simulink model "my_svpwm_controller"  (R2020a)
settings: Solver=VariableStepAuto  StartTime=0.0  StopTime=0.05  FixedStep=10e-6  MaxStep=0.00001  RelTol=1e-3  EnableMultiTasking=on
InitFcn:
  | f = 50;
libraries: dsparch4 x3, simulink x1, powerlib x1
settings Model: Creator=Administrator  LastModifiedBy=DELL
settings DataIOCC: LimitDataPoints=on  SaveFormat=Array  SignalLoggingSaveFormat=ModelDataLogs  ReturnWorkspaceOutputs=off
settings OptimizationCC: ExpressionDepthLimit=2147483647  InitFltsAndDblsToZero=on  LifeSpan=inf
settings DebuggingCC: SaveWithParameterizedLinksMsg=none  UnderspecifiedInitializationDetection=Classic  MergeDetectMultiDrivingBlocksExec=none  SignalResolutionControl=TryResolveAllWithWarning  SolverPrmCheckMsg=warning  MultiTaskDSMMsg=warning  MultiTaskCondExecSysMsg=none  FcnCallInpInsideContextMsg=warning  StateNameClashWarn=warning  SFUnexpectedBacktrackingDiag=warning  SFNoUnconditionalDefaultTransitionDiag=warning  ArithmeticOperatorsInVariantConditions=warning
settings HardwareCC: ProdBitPerPointer=32  ProdBitPerSizeT=32  ProdBitPerPtrDiffT=32  ProdLargestAtomicFloat=None  ProdIntDivRoundTo=Undefined  ProdEndianess=Unspecified  ProdWordSize=32  ProdHWDeviceType=32-bit Generic
settings ModelReferenceCC: PropagateSignalLabelsOutOfModel=off
settings SFSimCC: SimUseLocalCustomCode=off  CustomCodeUndefinedFunction=UseInterfaceOnly
settings RTWCC: RTWUseLocalCustomCode=off
settings CodeAppCC: StateflowObjectComments=on
settings GRTTargetCC: TargetFcnLib=ansi_tfl_tmw.mat  TargetLangStandard=C89/C90 (ANSI)  CombineOutputUpdateFcns=off  GRTInterface=on
settings ConfigComp: CovMetricSettings=dw  CovHtmlReporting=on  CovSaveCumulativeToWorkspaceVar=on  CovSaveSingleToWorkspaceVar=on  CovExternalEMLEnable=off

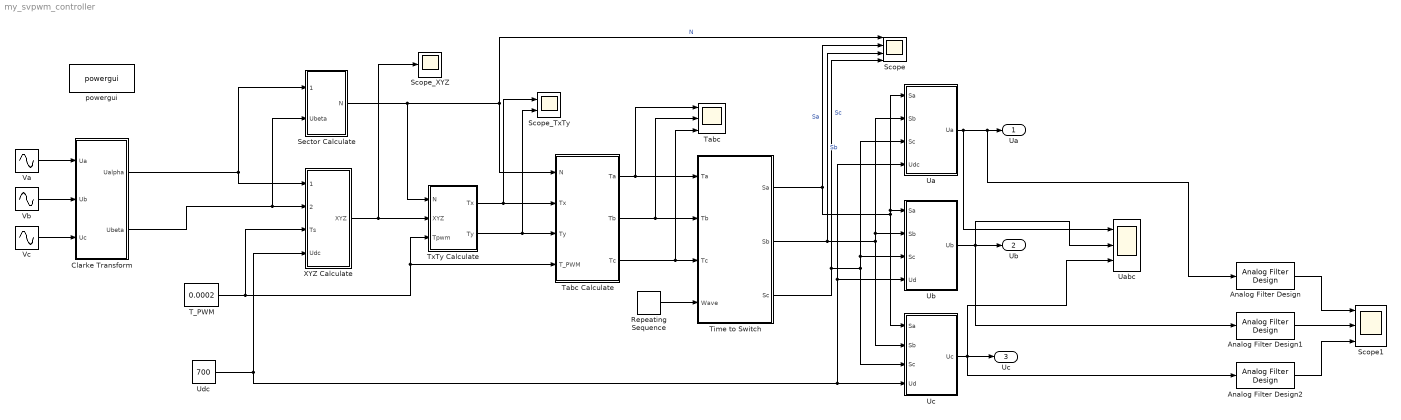
== system my_svpwm_controller ==
  Analog Filter Design : dsparch4/Analog Filter Design  method=Butterworth  filttype=Lowpass  N=4  Wlo=5*2*pi*f  Whi=80  Rp=2  Rs=40
  Analog Filter Design1 : dsparch4/Analog Filter Design  method=Butterworth  filttype=Lowpass  N=4  Wlo=5*2*pi*f  Whi=80  Rp=2  Rs=40
  Analog Filter Design2 : dsparch4/Analog Filter Design  method=Butterworth  filttype=Lowpass  N=4  Wlo=5*2*pi*f  Whi=80  Rp=2  Rs=40
  Clarke Transform : MATLAB Function  TreatAsAtomicUnit=on
  Repeating Sequence : simulink/Sources/Repeating Sequence  rep_seq_t=[0 1/10000 1/5000]  rep_seq_y=[0 1/10000 0]
  Scope : Scope  NumInputPorts=4
  Scope1 : Scope  NumInputPorts=3
  Scope_TxTy : Scope  NumInputPorts=2
  Scope_XYZ : Scope
  Sector Calculate : Subsystem
  T_PWM : Constant  Value=0.0002
  Tabc : Scope  NumInputPorts=3
  Tabc Calculate : Subsystem
  Time to Switch : Subsystem
  TxTy Calculate : Subsystem
  "Ua " : Subsystem
  Uabc : Scope  NumInputPorts=3
  "Ub " : Subsystem
  "Uc  " : Subsystem
  Udc : Constant  Value=700
  Va : Sin  Amplitude=200  Frequency=2*pi*f  SampleTime=0
  Vb : Sin  Amplitude=200  Frequency=2*pi*f  Phase=-2*pi/3  SampleTime=0
  Vc : Sin  Amplitude=200  Frequency=2*pi*f  Phase=-4*pi/3  SampleTime=0
  XYZ Calculate : Subsystem
  powergui : powerlib/powergui  Priority=1  SimulationMode=Discrete  SampleTime=1e-6  frequency=60  Iterations=50  frequencyindice=0  Pbase=100e6  ErrMax=1e-4  UnitsV=V  UnitsW=MW  buscounter=0  FunctionMessages=off  echomessages=off  EnableUseOfTLC=off  CurrentSourceSwitches=off  DisableSnubberDevices=off  DisableRonSwitches=off  DisableVfSwitches=off  DisplayEquations=off  AutomaticDiscreteSolvers=off  SolverType=Tustin/Backward Euler (TBE)  Interpol=off  ExternalGateDelay=off  methode=off  Ts=100  x0status=blocks  SPID=off  SwTol=0  HookPort=off  NonlinearTolerance=1e-4  nMaxIteration=100  ContinueOnMaxIteration=off  RestoreLinks=warning  ResistiveCurrentMeasurement=off  Frange=[0:2:500]  Ylog=off  Xlog=on  ShowGrid=off  save=off  variable=ZData  structure=aa3  ZoomFFT=off  StartTime=0.5  cycles=19  DisplayStyle=1  fundamental=50  FreqAxis=off  MaxFrequency=770  frequencyindicesteady=1  RmsSteady=1  display=off
  Ua : Outport  VectorParamsAs1DForOutWhenUnconnected=off
  Ub : Outport  Port=2  VectorParamsAs1DForOutWhenUnconnected=off
  Uc : Outport  Port=3  VectorParamsAs1DForOutWhenUnconnected=off
  wires:
  Clarke Transform/1(Ualpha) -> Sector Calculate/1(Ualpha), XYZ Calculate/1(Ualpha)
  Clarke Transform/2(Ubeta) -> Sector Calculate/2(Ubeta), XYZ Calculate/2(Ubeta)
  XYZ Calculate/1(XYZ) -> Scope_XYZ/1, TxTy Calculate/2(XYZ)
  TxTy Calculate/1(Tx) -> Scope_TxTy/1, Tabc Calculate/2(Tx)
  TxTy Calculate/2(Ty) -> Scope_TxTy/2, Tabc Calculate/3(Ty)
  Sector Calculate/1("N ") -> Scope/1, Tabc Calculate/1(N), TxTy Calculate/1(N)  "N"
  Repeating Sequence/1 -> Time to Switch/4(Wave)
  Time to Switch/1(Sa) -> Scope/2, "Ua "/1(Sa), "Ub "/1(Sa), "Uc  "/1("Sa ")  "Sa"
  Time to Switch/2(Sb) -> Scope/3, "Ua "/2(Sb), "Ub "/2(Sb), "Uc  "/2(Sb)  "Sb"
  Time to Switch/3(Sc) -> Scope/4, "Ua "/3(Sc), "Ub "/3(Sc), "Uc  "/3(Sc)  "Sc"
  "Ua "/1(Ua) -> Uabc/1, Analog Filter Design/1, Ua/1
  "Ub "/1(Ub) -> Analog Filter Design1/1, Uabc/2, Ub/1
  "Uc  "/1(Uc) -> Analog Filter Design2/1, Uc/1, Uabc/3
  T_PWM/1 -> Tabc Calculate/4(T_PWM), TxTy Calculate/3(Tpwm), XYZ Calculate/3(Ts)
  Udc/1 -> XYZ Calculate/4(Udc), "Uc  "/4(Ud), "Ua "/4(Udc), "Ub "/4(Ud)
  Vc/1 -> Clarke Transform/3(Uc)
  Vb/1 -> Clarke Transform/2(Ub)
  Va/1 -> Clarke Transform/1(Ua)
  Tabc Calculate/1(Ta) -> Time to Switch/1(Ta), Tabc/1
  Tabc Calculate/2(Tb) -> Time to Switch/2(Tb), Tabc/2
  Tabc Calculate/3(Tc) -> Tabc/3, Time to Switch/3(Tc)
  Analog Filter Design2/1 -> Scope1/3
  Analog Filter Design1/1 -> Scope1/2
  Analog Filter Design/1 -> Scope1/1

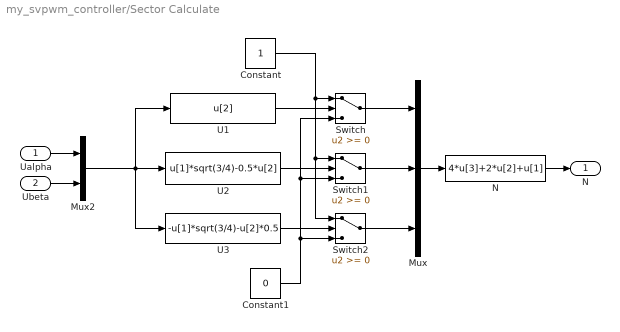
== system my_svpwm_controller/Sector Calculate ==
  Ualpha : Inport
  Ubeta : Inport  Port=2
  Constant : Constant
  Constant1 : Constant  Value=0
  Mux : Mux  Inputs=3
  Mux2 : Mux  Inputs=2
  N : Fcn  Expr=4*u[3]+2*u[2]+u[1]
  Switch : Switch
  Switch1 : Switch
  Switch2 : Switch
  U1 : Fcn  Expr=u[2]
  U2 : Fcn  Expr=u[1]*sqrt(3/4)-0.5*u[2]
  U3 : Fcn  Expr=-u[1]*sqrt(3/4)-u[2]*0.5
  "N " : Outport  VectorParamsAs1DForOutWhenUnconnected=off
  wires:
  Switch2/1 -> Mux/3
  Switch/1 -> Mux/1
  Ualpha/1 -> Mux2/1
  Ubeta/1 -> Mux2/2
  Mux2/1 -> U1/1, U3/1, U2/1
  U1/1 -> Switch/2
  U2/1 -> Switch1/2
  U3/1 -> Switch2/2
  Constant/1 -> Switch/1, Switch2/1, Switch1/1
  Constant1/1 -> Switch/3, Switch1/3, Switch2/3
  Switch1/1 -> Mux/2
  Mux/1 -> N/1
  N/1 -> "N "/1

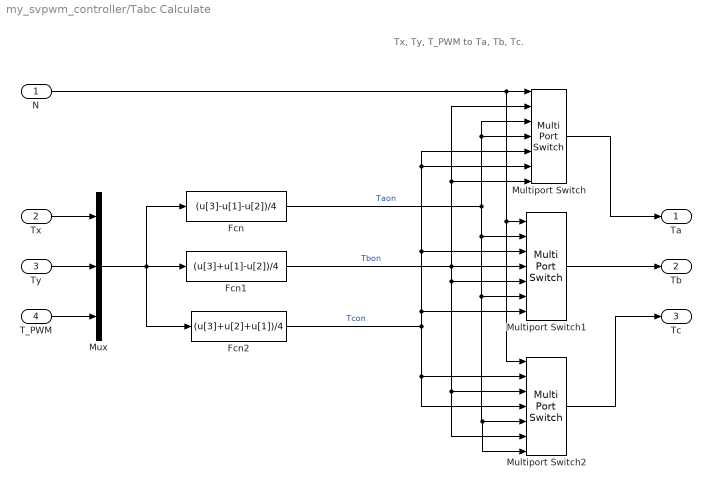
== system my_svpwm_controller/Tabc Calculate ==
  note: Tx, Ty, T_PWM to Ta, Tb, Tc.
  N : Inport
  Tx : Inport  Port=2
  Ty : Inport  Port=3
  T_PWM : Inport  Port=4
  Fcn : Fcn  Expr=(u[3]-u[1]-u[2])/4
  Fcn1 : Fcn  Expr=(u[3]+u[1]-u[2])/4
  Fcn2 : Fcn  Expr=(u[3]+u[2]+u[1])/4
  Multiport Switch : MultiPortSwitch  Inputs=6
  Multiport Switch1 : MultiPortSwitch  Inputs=6
  Multiport Switch2 : MultiPortSwitch  Inputs=6
  Mux : Mux  Inputs=3
  Ta : Outport
  Tb : Outport  Port=2
  Tc : Outport  Port=3
  wires:
  Mux/1 -> Fcn2/1, Fcn/1, Fcn1/1
  T_PWM/1 -> Mux/3
  Ty/1 -> Mux/2
  Tx/1 -> Mux/1
  Multiport Switch2/1 -> Tc/1
  Multiport Switch1/1 -> Tb/1
  Multiport Switch/1 -> Ta/1
  Fcn/1 -> Multiport Switch/3, Multiport Switch/4, Multiport Switch1/6, Multiport Switch2/5, Multiport Switch2/7, Multiport Switch1/2  "Taon"
  Fcn1/1 -> Multiport Switch1/5, Multiport Switch2/3, Multiport Switch2/6, Multiport Switch1/4, Multiport Switch/7, Multiport Switch/2  "Tbon"
  Fcn2/1 -> Multiport Switch/5, Multiport Switch/6, Multiport Switch1/3, Multiport Switch1/7, Multiport Switch2/2, Multiport Switch2/4  "Tcon"
  N/1 -> Multiport Switch2/1, Multiport Switch1/1, Multiport Switch/1

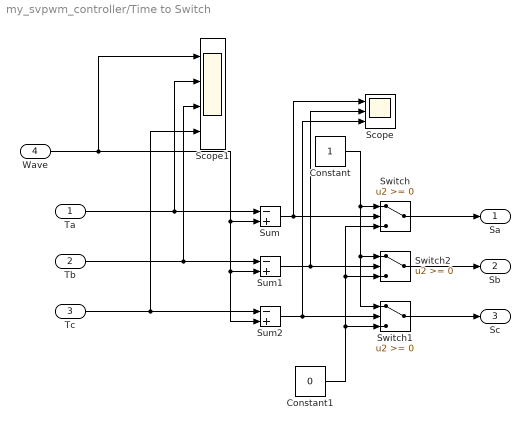
== system my_svpwm_controller/Time to Switch ==
  Ta : Inport
  Tb : Inport  Port=2
  Tc : Inport  Port=3
  Wave : Inport  Port=4
  Constant : Constant
  Constant1 : Constant  Value=0
  Scope : Scope  NumInputPorts=3
  Scope1 : Scope  NumInputPorts=4
  Sum : Sum  Inputs=-+
  Sum1 : Sum  Inputs=-+
  Sum2 : Sum  Inputs=-+
  Switch : Switch  SaturateOnIntegerOverflow=on
  Switch1 : Switch  SaturateOnIntegerOverflow=on
  Switch2 : Switch  SaturateOnIntegerOverflow=on
  Sa : Outport  VectorParamsAs1DForOutWhenUnconnected=off
  Sb : Outport  Port=2  VectorParamsAs1DForOutWhenUnconnected=off
  Sc : Outport  Port=3  VectorParamsAs1DForOutWhenUnconnected=off
  wires:
  Switch1/1 -> Sc/1
  Switch2/1 -> Sb/1
  Switch/1 -> Sa/1
  Constant1/1 -> Switch1/3, Switch2/3, Switch/3
  Constant/1 -> Switch/1, Switch2/1, Switch1/1
  Sum2/1 -> Switch1/2, Scope/3
  Sum1/1 -> Scope/2, Switch2/2
  Sum/1 -> Scope/1, Switch/2
  Tc/1 -> Sum2/1, Scope1/4
  Tb/1 -> Scope1/3, Sum1/1
  Ta/1 -> Scope1/2, Sum/1
  Wave/1 -> Scope1/1, Sum1/2, Sum2/2, Sum/2

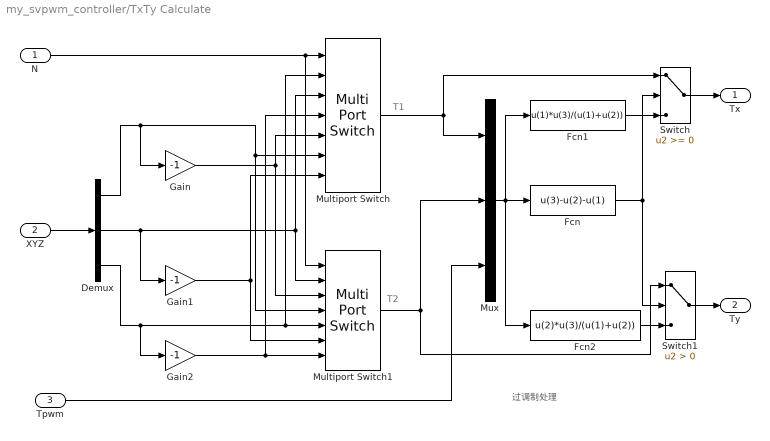
== system my_svpwm_controller/TxTy Calculate ==
  note: 过调制处理
  note: T1
  note: T2
  N : Inport
  XYZ : Inport  Port=2
  Tpwm : Inport  Port=3
  Demux : Demux  Outputs=3
  Fcn : Fcn  Expr=u(3)-u(2)-u(1)
  Fcn1 : Fcn  Expr=u(1)*u(3)/(u(1)+u(2))
  Fcn2 : Fcn  Expr=u(2)*u(3)/(u(1)+u(2))
  Gain : Gain  Gain=-1
  Gain1 : Gain  Gain=-1
  Gain2 : Gain  Gain=-1
  Multiport Switch : MultiPortSwitch  Inputs=6
  Multiport Switch1 : MultiPortSwitch  Inputs=6
  Mux : Mux  Inputs=3
  Switch : Switch
  Switch1 : Switch  Criteria=u2 > Threshold
  Tx : Outport  VectorParamsAs1DForOutWhenUnconnected=off
  Ty : Outport  Port=2  VectorParamsAs1DForOutWhenUnconnected=off
  wires:
  Tpwm/1 -> Mux/3
  XYZ/1 -> Demux/1
  Switch1/1 -> Ty/1
  Switch/1 -> Tx/1
  Fcn2/1 -> Switch1/3
  Fcn1/1 -> Switch/3
  Fcn/1 -> Switch/2, Switch1/2
  Mux/1 -> Fcn1/1, Fcn/1, Fcn2/1
  Multiport Switch/1 -> Switch/1, Mux/1
  Multiport Switch1/1 -> Switch1/1, Mux/2
  N/1 -> Multiport Switch/1, Multiport Switch1/1
  Demux/2 -> Multiport Switch/3, Multiport Switch1/2, Gain1/1
  Demux/3 -> Multiport Switch1/5, Multiport Switch/2, Gain2/1
  Demux/1 -> Multiport Switch/6, Multiport Switch1/4, Gain/1
  Gain/1 -> Multiport Switch1/3, Multiport Switch/5
  Gain2/1 -> Multiport Switch/4, Multiport Switch1/7
  Gain1/1 -> Multiport Switch1/6, Multiport Switch/7

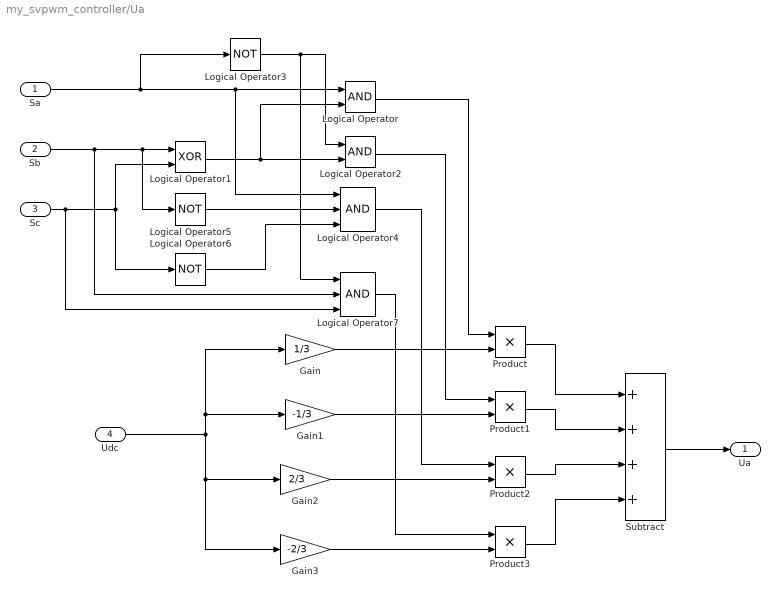
== system my_svpwm_controller/Ua  ==
  Sa : Inport
  Sb : Inport  Port=2
  Sc : Inport  Port=3
  Udc : Inport  Port=4
  Gain : Gain  Gain=1/3
  Gain1 : Gain  Gain=-1/3
  Gain2 : Gain  Gain=2/3
  Gain3 : Gain  Gain=-2/3
  Logical Operator : Logic  AllPortsSameDT=off  OutDataTypeStr=boolean
  Logical Operator1 : Logic  Operator=XOR  AllPortsSameDT=off  OutDataTypeStr=boolean
  Logical Operator2 : Logic  AllPortsSameDT=off  OutDataTypeStr=boolean
  Logical Operator3 : Logic  Operator=NOT  AllPortsSameDT=off  OutDataTypeStr=boolean
  Logical Operator4 : Logic  Inputs=3  AllPortsSameDT=off  OutDataTypeStr=boolean
  Logical Operator5 : Logic  Operator=NOT  AllPortsSameDT=off  OutDataTypeStr=boolean
  Logical Operator6 : Logic  Operator=NOT  AllPortsSameDT=off  OutDataTypeStr=boolean
  Logical Operator7 : Logic  Inputs=3  AllPortsSameDT=off  OutDataTypeStr=boolean
  Product{,1..3} (4 alike) : Product  RndMeth=Zero
  Subtract : Sum  Inputs=++++
  Ua : Outport  VectorParamsAs1DForOutWhenUnconnected=off
  wires:
  Udc/1 -> Gain3/1, Gain2/1, Gain1/1, Gain/1
  Gain/1 -> Product/2
  Gain1/1 -> Product1/2
  Gain2/1 -> Product2/2
  Gain3/1 -> Product3/2
  Product/1 -> Subtract/1
  Product1/1 -> Subtract/2
  Product2/1 -> Subtract/3
  Product3/1 -> Subtract/4
  Subtract/1 -> Ua/1
  Logical Operator/1 -> Product/1
  Sa/1 -> Logical Operator4/1, Logical Operator/1, Logical Operator3/1
  Sb/1 -> Logical Operator5/1, Logical Operator1/1, Logical Operator7/2
  Sc/1 -> Logical Operator7/3, Logical Operator1/2, Logical Operator6/1
  Logical Operator1/1 -> Logical Operator/2, Logical Operator2/2
  Logical Operator2/1 -> Product1/1
  Logical Operator3/1 -> Logical Operator2/1, Logical Operator7/1
  Logical Operator4/1 -> Product2/1
  Logical Operator5/1 -> Logical Operator4/2
  Logical Operator6/1 -> Logical Operator4/3
  Logical Operator7/1 -> Product3/1

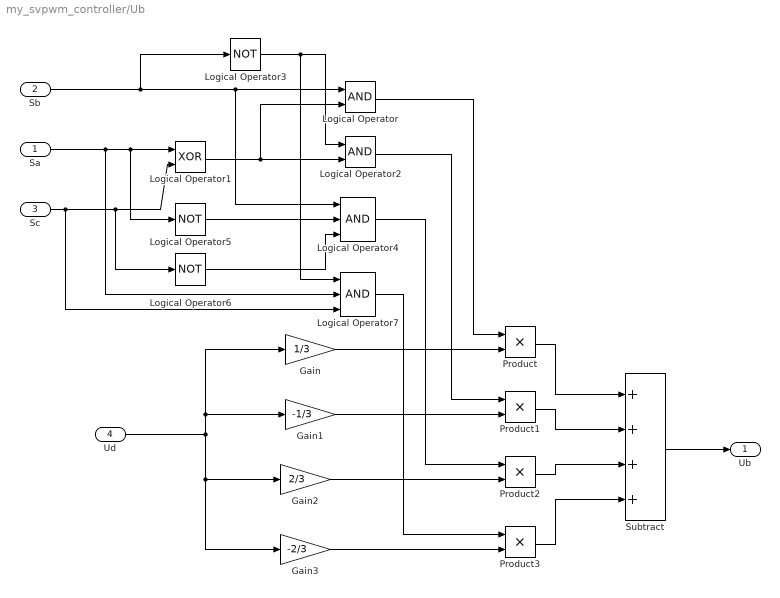
== system my_svpwm_controller/Ub  ==
  Sa : Inport
  Sb : Inport  Port=2
  Sc : Inport  Port=3
  Ud : Inport  Port=4
  Gain : Gain  Gain=1/3
  Gain1 : Gain  Gain=-1/3
  Gain2 : Gain  Gain=2/3
  Gain3 : Gain  Gain=-2/3
  Logical Operator : Logic  AllPortsSameDT=off  OutDataTypeStr=boolean
  Logical Operator1 : Logic  Operator=XOR  AllPortsSameDT=off  OutDataTypeStr=boolean
  Logical Operator2 : Logic  AllPortsSameDT=off  OutDataTypeStr=boolean
  Logical Operator3 : Logic  Operator=NOT  AllPortsSameDT=off  OutDataTypeStr=boolean
  Logical Operator4 : Logic  Inputs=3  AllPortsSameDT=off  OutDataTypeStr=boolean
  Logical Operator5 : Logic  Operator=NOT  AllPortsSameDT=off  OutDataTypeStr=boolean
  Logical Operator6 : Logic  Operator=NOT  AllPortsSameDT=off  OutDataTypeStr=boolean
  Logical Operator7 : Logic  Inputs=3  AllPortsSameDT=off  OutDataTypeStr=boolean
  Product{,1..3} (4 alike) : Product  RndMeth=Zero
  Subtract : Sum  Inputs=++++
  Ub : Outport  VectorParamsAs1DForOutWhenUnconnected=off
  wires:
  Ud/1 -> Gain3/1, Gain2/1, Gain1/1, Gain/1
  Gain/1 -> Product/2
  Gain1/1 -> Product1/2
  Gain2/1 -> Product2/2
  Gain3/1 -> Product3/2
  Product/1 -> Subtract/1
  Product1/1 -> Subtract/2
  Product2/1 -> Subtract/3
  Product3/1 -> Subtract/4
  Subtract/1 -> Ub/1
  Logical Operator/1 -> Product/1
  Sb/1 -> Logical Operator4/1, Logical Operator/1, Logical Operator3/1
  Sa/1 -> Logical Operator7/2, Logical Operator5/1, Logical Operator1/1
  Sc/1 -> Logical Operator7/3, Logical Operator1/2, Logical Operator6/1
  Logical Operator1/1 -> Logical Operator/2, Logical Operator2/2
  Logical Operator2/1 -> Product1/1
  Logical Operator3/1 -> Logical Operator2/1, Logical Operator7/1
  Logical Operator4/1 -> Product2/1
  Logical Operator5/1 -> Logical Operator4/2
  Logical Operator6/1 -> Logical Operator4/3
  Logical Operator7/1 -> Product3/1

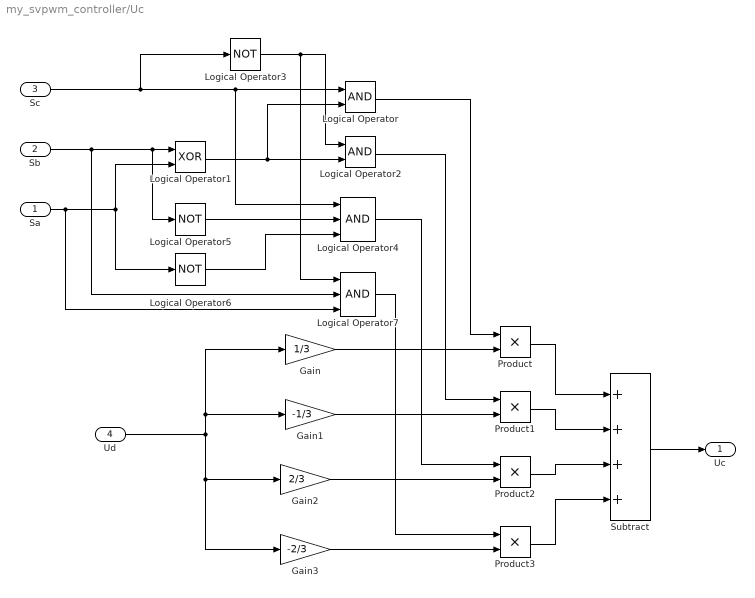
== system my_svpwm_controller/Uc   ==
  "Sa " : Inport
  Sb : Inport  Port=2
  Sc : Inport  Port=3
  Ud : Inport  Port=4
  Gain : Gain  Gain=1/3
  Gain1 : Gain  Gain=-1/3
  Gain2 : Gain  Gain=2/3
  Gain3 : Gain  Gain=-2/3
  Logical Operator : Logic  AllPortsSameDT=off  OutDataTypeStr=boolean
  Logical Operator1 : Logic  Operator=XOR  AllPortsSameDT=off  OutDataTypeStr=boolean
  Logical Operator2 : Logic  AllPortsSameDT=off  OutDataTypeStr=boolean
  Logical Operator3 : Logic  Operator=NOT  AllPortsSameDT=off  OutDataTypeStr=boolean
  Logical Operator4 : Logic  Inputs=3  AllPortsSameDT=off  OutDataTypeStr=boolean
  Logical Operator5 : Logic  Operator=NOT  AllPortsSameDT=off  OutDataTypeStr=boolean
  Logical Operator6 : Logic  Operator=NOT  AllPortsSameDT=off  OutDataTypeStr=boolean
  Logical Operator7 : Logic  Inputs=3  AllPortsSameDT=off  OutDataTypeStr=boolean
  Product{,1..3} (4 alike) : Product  RndMeth=Zero
  Subtract : Sum  Inputs=++++
  Uc : Outport  VectorParamsAs1DForOutWhenUnconnected=off
  wires:
  Ud/1 -> Gain3/1, Gain2/1, Gain1/1, Gain/1
  Gain/1 -> Product/2
  Gain1/1 -> Product1/2
  Gain2/1 -> Product2/2
  Gain3/1 -> Product3/2
  Product/1 -> Subtract/1
  Product1/1 -> Subtract/2
  Product2/1 -> Subtract/3
  Product3/1 -> Subtract/4
  Subtract/1 -> Uc/1
  Logical Operator/1 -> Product/1
  Sc/1 -> Logical Operator4/1, Logical Operator/1, Logical Operator3/1
  Sb/1 -> Logical Operator5/1, Logical Operator1/1, Logical Operator7/2
  "Sa "/1 -> Logical Operator7/3, Logical Operator1/2, Logical Operator6/1
  Logical Operator1/1 -> Logical Operator/2, Logical Operator2/2
  Logical Operator2/1 -> Product1/1
  Logical Operator3/1 -> Logical Operator2/1, Logical Operator7/1
  Logical Operator4/1 -> Product2/1
  Logical Operator5/1 -> Logical Operator4/2
  Logical Operator6/1 -> Logical Operator4/3
  Logical Operator7/1 -> Product3/1

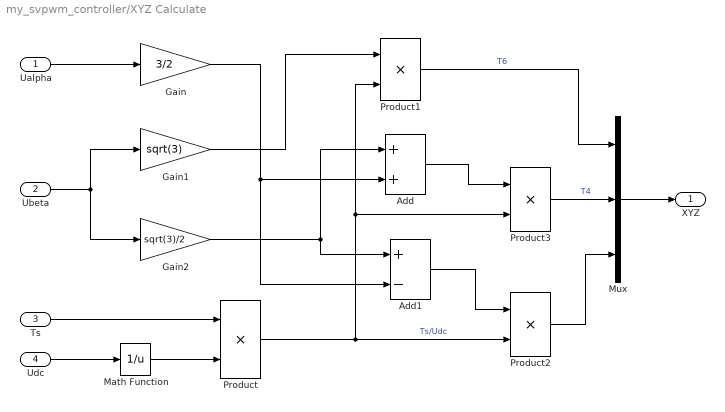
== system my_svpwm_controller/XYZ Calculate ==
  Ualpha : Inport
  Ubeta : Inport  Port=2
  Ts : Inport  Port=3
  Udc : Inport  Port=4
  Add : Sum
  Add1 : Sum  Inputs=+-
  Gain : Gain  Gain=3/2
  Gain1 : Gain  Gain=sqrt(3)
  Gain2 : Gain  Gain=sqrt(3)/2
  Math Function : Math  Operator=reciprocal  SignedPower=on  SaturateOnIntegerOverflow=on
  Mux : Mux  Inputs=3
  Product{,1..3} (4 alike) : Product  RndMeth=Zero
  XYZ : Outport  VectorParamsAs1DForOutWhenUnconnected=off
  wires:
  Mux/1 -> XYZ/1
  Product1/1 -> Mux/1  "T6"
  Product3/1 -> Mux/2  "T4"
  Product2/1 -> Mux/3
  Ualpha/1 -> Gain/1
  Ubeta/1 -> Gain2/1, Gain1/1
  Udc/1 -> Math Function/1
  Math Function/1 -> Product/2
  Ts/1 -> Product/1
  Gain1/1 -> Product1/1
  Product/1 -> Product2/2, Product1/2, Product3/2  "Ts/Udc"
  Gain/1 -> Add1/2, Add/2
  Gain2/1 -> Add/1, Add1/1
  Add1/1 -> Product2/1
  Add/1 -> Product3/1

== matlab function my_svpwm_controller/Clarke Transform ==
  data: Ualpha output; Ubeta output; Ua input; Ub input; Uc input
function [Ualpha, Ubeta]= fcn(Ua, Ub, Uc)

% m = 2/3

U = 2/3 * [1 -0.5 -0.5; 0 sqrt(3)/2 -sqrt(3)/2] * [Ua; Ub; Uc];
Ualpha = U(1);
Ubeta = U(2);

end
